simulink model "RTP_V39"  (R2020b)
settings: Solver=ode4  StartTime=0.0  StopTime=40  FixedStep=0.0001  RelTol=1e-3
settings Model: Creator=barac  LastModifiedBy=barac

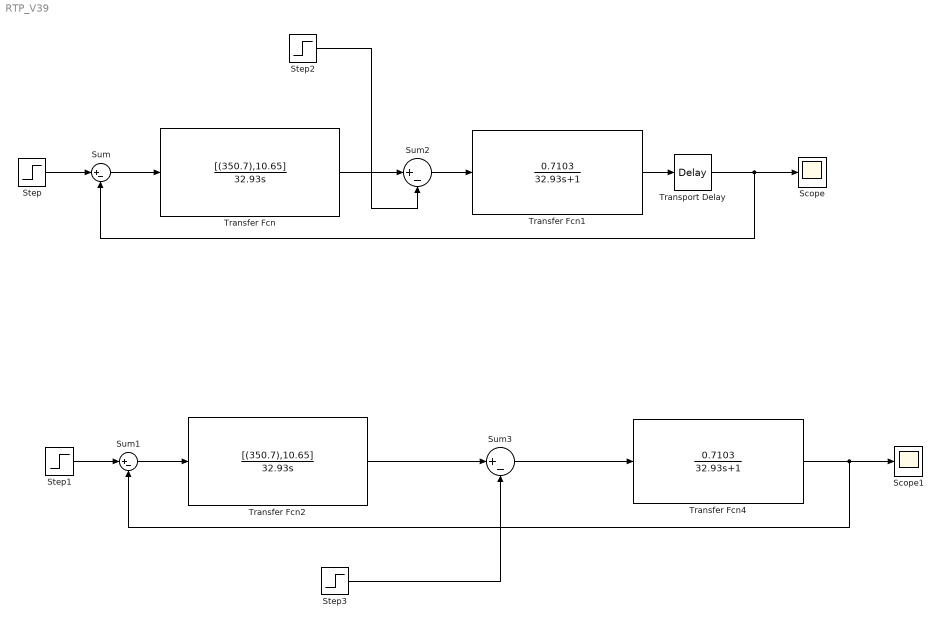
== system RTP_V39 ==
  Scope : Scope
  Scope1 : Scope
  Step : Step  SampleTime=0
  Step1 : Step  SampleTime=0
  Step2 : Step  After=0.1  SampleTime=0
  Step3 : Step  SampleTime=0
  Sum{,1..3} (4 alike) : Sum  Inputs=|+-
  Transfer Fcn : TransferFcn  Numerator=[(350.7),10.65]  Denominator=[32.93 0]
  Transfer Fcn1 : TransferFcn  Numerator=[0.7103]  Denominator=[32.93 1]
  Transfer Fcn2 : TransferFcn  Numerator=[(350.7),10.65]  Denominator=[32.93 0]
  Transfer Fcn4 : TransferFcn  Numerator=[0.7103]  Denominator=[32.93 1]
  Transport Delay : TransportDelay
  wires:
  Transfer Fcn1/1 -> Transport Delay/1
  Step/1 -> Sum/1
  Sum/1 -> Transfer Fcn/1
  Transfer Fcn2/1 -> Sum3/1
  Sum3/1 -> Transfer Fcn4/1
  Step1/1 -> Sum1/1
  Sum1/1 -> Transfer Fcn2/1
  Transfer Fcn/1 -> Sum2/1
  Transport Delay/1 -> Sum/2, Scope/1
  Step2/1 -> Sum2/2
  Step3/1 -> Sum3/2
  Sum2/1 -> Transfer Fcn1/1
  Transfer Fcn4/1 -> Scope1/1, Sum1/2
